simulink model "CHB_1phase"  (R2015a)
settings: Solver=ode45  StartTime=0.0  StopTime=10.0  MaxStep=0.000001  MinStep=0.0000001  RelTol=1e-3
libraries: powerlib x18, simulink x1
settings Model: Creator=hp  LastModifiedBy=hp

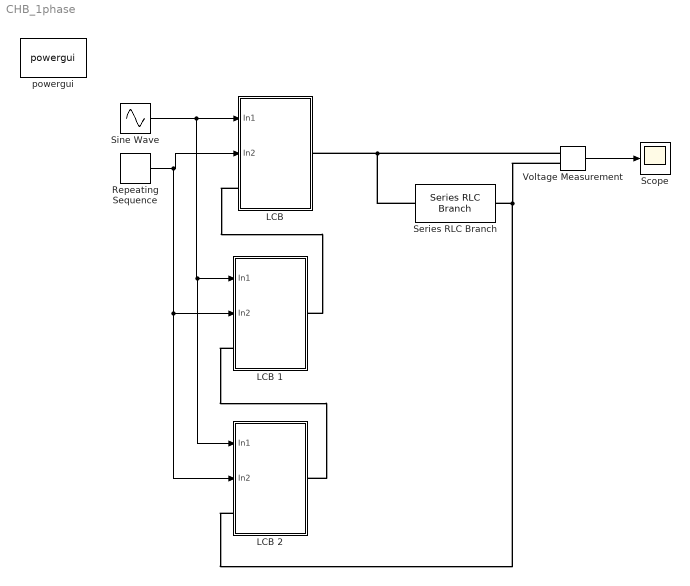
== system CHB_1phase ==
  "LCB " : Subsystem
  LCB 1 : Subsystem
  LCB 2 : Subsystem
  Repeating Sequence : simulink/Sources/Repeating Sequence  rep_seq_t=[0 0.25 0.5 0.75 1]/1000  rep_seq_y=[0 1 0 -1 0]
  Scope : Scope
      settings: YMin=-80  YMax=80
  Series RLC Branch : powerlib/Elements/Series RLC Branch  LConnTagsString=__new0  RConnTagsString=__new0  BranchType=RLC  Resistance=1  Inductance=0  SetiL0=off  InitialCurrent=0  Capacitance=0  Setx0=off  InitialVoltage=0  Measurements=None
  Sine Wave : Sin  Amplitude=0.95  Frequency=2*pi*50  SampleTime=0
  Voltage Measurement : powerlib/Measurements/Voltage Measurement  PhasorSimulation=off  OutputType=Complex  PSBequivalent=0
  powergui : powerlib/powergui  Priority=1  SimulationMode=Continuous  SolverType=Tustin/Backward Euler (TBE)  SampleTime=50e-6  frequency=60  SPID=off  DisableSnubberDevices=off  DisableRonSwitches=off  DisableVfSwitches=off  SwTol=0  DisplayEquations=off  Interpol=off  methode=off  Ts=100  FunctionMessages=off  echomessages=off  HookPort=off  EnableUseOfTLC=off  x0status=blocks  frequencyindice=0  Pbase=100e6  ErrMax=1e-4  Iterations=50  UnitsV=kV  UnitsW=MW  buscounter=0  RestoreLinks=warning  ResistiveCurrentMeasurement=off  Frange=[0:2:500]  Ylog=off  Xlog=on  ShowGrid=off  save=off  variable=ZData  structure=0  ZoomFFT=off  StartTime=0.0  cycles=1  DisplayStyle=1  fundamental=60  FreqAxis=off  MaxFrequency=1000  frequencyindicesteady=1  RmsSteady=1  display=off
  wires:
  Voltage Measurement/1 -> Scope/1
  Sine Wave/1 -> LCB 2/1(In1), LCB 1/1(In1), "LCB "/1(In1)
  Repeating Sequence/1 -> LCB 2/2(In2), LCB 1/2(In2), "LCB "/2(In2)
  connections:
  "LCB "/LConn1 -- LCB 1/RConn1
  Series RLC Branch/LConn1 -- "LCB "/RConn1 -- Voltage Measurement/LConn1
  Voltage Measurement/LConn2 -- LCB 2/LConn1 -- Series RLC Branch/RConn1
  LCB 1/LConn1 -- LCB 2/RConn1

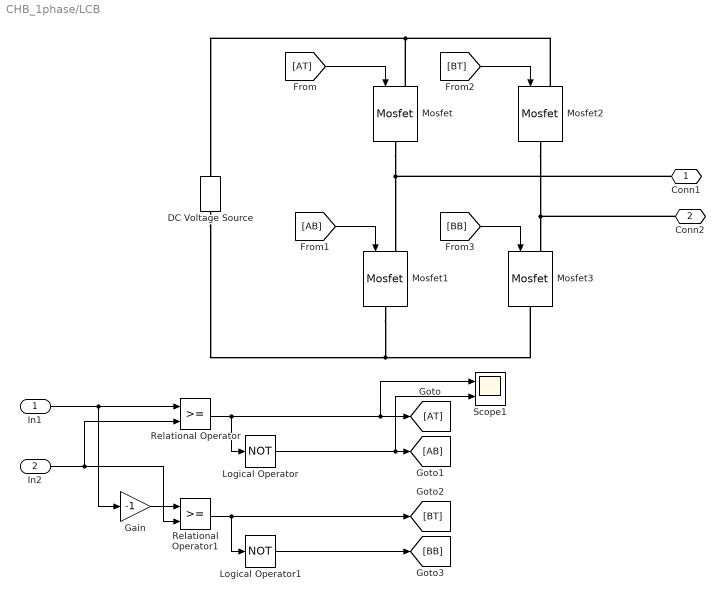
== system CHB_1phase/LCB  ==
  In1 : Inport
  In2 : Inport  Port=2
  DC Voltage Source : powerlib/Electrical Sources/DC Voltage Source  Amplitude=100  Measurements=None
  Gain : Gain  Gain=-1
  Logical Operator : Logic  Operator=NOT  Inputs=1  AllPortsSameDT=off  OutDataTypeStr=boolean
  Logical Operator1 : Logic  Operator=NOT  Inputs=1  AllPortsSameDT=off  OutDataTypeStr=boolean
  Mosfet{,1..3} (4 alike) : powerlib/Power Electronics/Mosfet  Ron=0.1  Lon=0  Rd=0.01  Vfd=0  IC=0  Rs=1e5  Cs=inf  Measurements=off
  Relational Operator : RelationalOperator  OutDataTypeStr=boolean
  Relational Operator1 : RelationalOperator  OutDataTypeStr=boolean
  Scope1 : Scope  NumInputPorts=2
      settings: YMin=-80~-5  YMax=80~5
  Conn1 : PMIOPort  Port=1  Side=Right
  Conn2 : PMIOPort  Port=2  Side=Left
  wires:
  Gain/1 -> Relational Operator1/1
  Relational Operator/1 -> Scope1/1, [AT], Logical Operator/1
  Logical Operator/1 -> Scope1/2, [AB]
  Relational Operator1/1 -> [BT], Logical Operator1/1
  Logical Operator1/1 -> [BB]
  [BB] -> Mosfet3/1
  [AB] -> Mosfet1/1
  [AT] -> Mosfet/1
  [BT] -> Mosfet2/1
  In2/1 -> Relational Operator1/2, Relational Operator/2
  In1/1 -> Gain/1, Relational Operator/1
  connections:
  Mosfet2/RConn1 -- Conn2/RConn1 -- Mosfet3/LConn1
  DC Voltage Source/LConn1 -- Mosfet1/RConn1 -- Mosfet3/RConn1
  Mosfet2/LConn1 -- Mosfet/LConn1 -- DC Voltage Source/RConn1
  Mosfet/RConn1 -- Conn1/RConn1 -- Mosfet1/LConn1

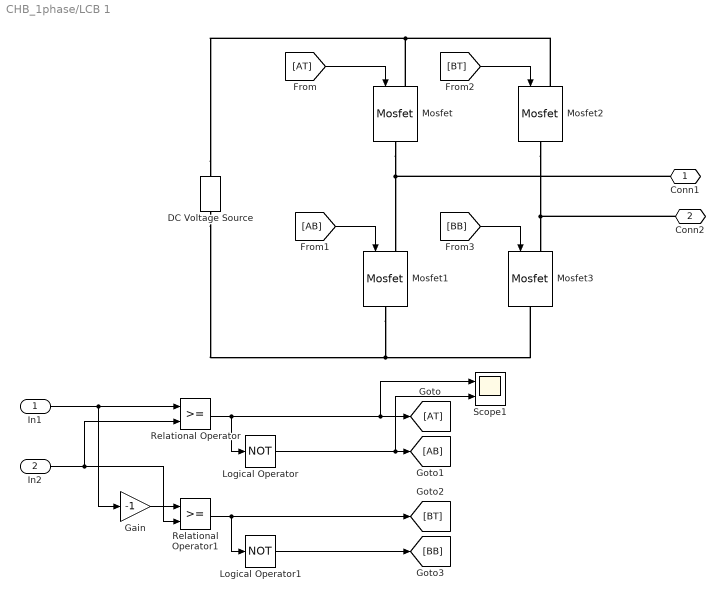
== system CHB_1phase/LCB 1 ==
  In1 : Inport
  In2 : Inport  Port=2
  DC Voltage Source : powerlib/Electrical Sources/DC Voltage Source  Amplitude=100  Measurements=None
  Gain : Gain  Gain=-1
  Logical Operator : Logic  Operator=NOT  Inputs=1  AllPortsSameDT=off  OutDataTypeStr=boolean
  Logical Operator1 : Logic  Operator=NOT  Inputs=1  AllPortsSameDT=off  OutDataTypeStr=boolean
  Mosfet{,1..3} (4 alike) : powerlib/Power Electronics/Mosfet  Ron=0.1  Lon=0  Rd=0.01  Vfd=0  IC=0  Rs=1e5  Cs=inf  Measurements=off
  Relational Operator : RelationalOperator  OutDataTypeStr=boolean
  Relational Operator1 : RelationalOperator  OutDataTypeStr=boolean
  Scope1 : Scope  NumInputPorts=2
      settings: YMin=-80~-5  YMax=80~5
  Conn1 : PMIOPort  Port=1  Side=Right
  Conn2 : PMIOPort  Port=2  Side=Left
  wires:
  Gain/1 -> Relational Operator1/1
  Relational Operator/1 -> Scope1/1, [AT], Logical Operator/1
  Logical Operator/1 -> Scope1/2, [AB]
  Relational Operator1/1 -> [BT], Logical Operator1/1
  Logical Operator1/1 -> [BB]
  [BB] -> Mosfet3/1
  [AB] -> Mosfet1/1
  [AT] -> Mosfet/1
  [BT] -> Mosfet2/1
  In2/1 -> Relational Operator1/2, Relational Operator/2
  In1/1 -> Gain/1, Relational Operator/1
  connections:
  Mosfet2/RConn1 -- Conn2/RConn1 -- Mosfet3/LConn1
  Mosfet3/RConn1 -- DC Voltage Source/LConn1 -- Mosfet1/RConn1
  DC Voltage Source/RConn1 -- Mosfet2/LConn1 -- Mosfet/LConn1
  Mosfet/RConn1 -- Mosfet1/LConn1 -- Conn1/RConn1

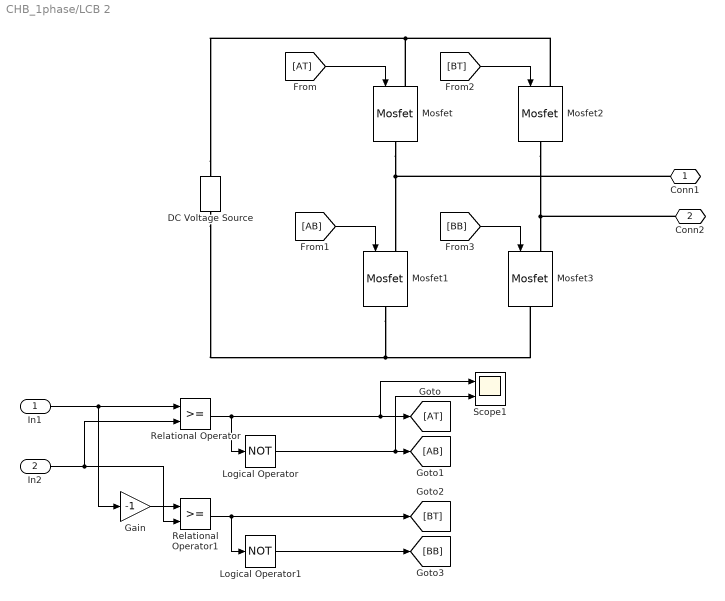
== system CHB_1phase/LCB 2 ==
  In1 : Inport
  In2 : Inport  Port=2
  DC Voltage Source : powerlib/Electrical Sources/DC Voltage Source  Amplitude=100  Measurements=None
  Gain : Gain  Gain=-1
  Logical Operator : Logic  Operator=NOT  Inputs=1  AllPortsSameDT=off  OutDataTypeStr=boolean
  Logical Operator1 : Logic  Operator=NOT  Inputs=1  AllPortsSameDT=off  OutDataTypeStr=boolean
  Mosfet{,1..3} (4 alike) : powerlib/Power Electronics/Mosfet  Ron=0.1  Lon=0  Rd=0.01  Vfd=0  IC=0  Rs=1e5  Cs=inf  Measurements=off
  Relational Operator : RelationalOperator  OutDataTypeStr=boolean
  Relational Operator1 : RelationalOperator  OutDataTypeStr=boolean
  Scope1 : Scope  NumInputPorts=2
      settings: YMin=-80~-5  YMax=80~5
  Conn1 : PMIOPort  Port=1  Side=Right
  Conn2 : PMIOPort  Port=2  Side=Left
  wires:
  Gain/1 -> Relational Operator1/1
  Relational Operator/1 -> Scope1/1, [AT], Logical Operator/1
  Logical Operator/1 -> Scope1/2, [AB]
  Relational Operator1/1 -> [BT], Logical Operator1/1
  Logical Operator1/1 -> [BB]
  [BB] -> Mosfet3/1
  [AB] -> Mosfet1/1
  [AT] -> Mosfet/1
  [BT] -> Mosfet2/1
  In2/1 -> Relational Operator1/2, Relational Operator/2
  In1/1 -> Gain/1, Relational Operator/1
  connections:
  Mosfet2/RConn1 -- Conn2/RConn1 -- Mosfet3/LConn1
  Mosfet3/RConn1 -- DC Voltage Source/LConn1 -- Mosfet1/RConn1
  DC Voltage Source/RConn1 -- Mosfet2/LConn1 -- Mosfet/LConn1
  Mosfet/RConn1 -- Mosfet1/LConn1 -- Conn1/RConn1
